simulink model "EPS_MILS"  (R2023a)
settings: Solver=ode23t  StartTime=0.0  StopTime=2  FixedStep=10e-6  RelTol=1e-3
undefined symbols (not defined in the file): Ion, Lithium
libraries: spsSeriesRLCBranchLib x5, spsVoltageMeasurementLib x3, spsPVArrayLib x2, spsCurrentMeasurementLib x2, spsPWMGeneratorDCDCLib x2, spsBatteryLib x1, spsDiodeLib x1, spsIGBTDiodeLib x1, sps_lib x1
settings Model: Creator=Ameya  LastModifiedBy=Ameya

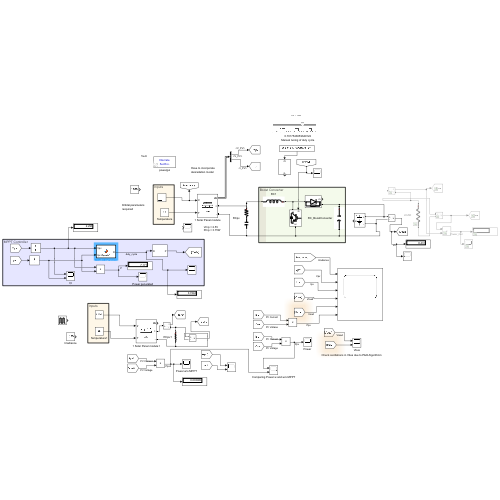
[thumbnail: Simulink's stored preview of the top-level diagram]
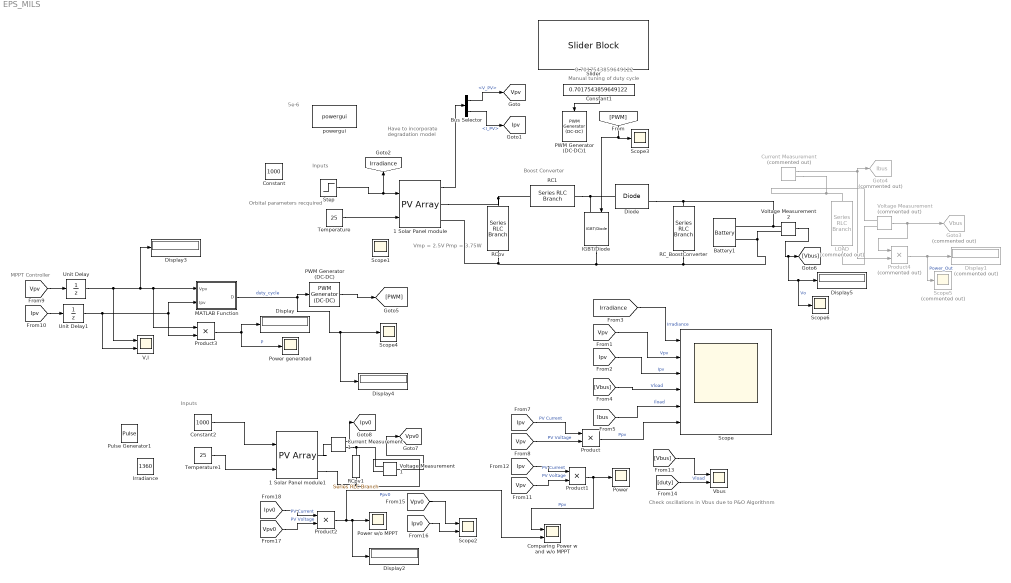
== system EPS_MILS ==
  note: 0.7017543859649122
  note: Manual tuning of duty cycle
  note: Vmp = 2.5V
      | Pmp = 3.75W
  note: 5e-6
  note: Check oscillations in Vbus due to P&O Algorithnm
  note: Boost Converter
  note: Orbital parameters recquired
  note: Have to incorporate degradation model
  note: Inputs
  note: MPPT Controller
  note: Inputs
  1 Solar Panel module : spsPVArrayLib/PV Array  Npar=1  Nser=1  PlotType=one module @ 25 deg.C & specified irradiances  S_vec="[ 1360 1000  500  100 ]"  Temp_C_vec="[ 45 25  ]"  ModuleName=User-defined  PlotWhenSelected=off  Pm=3.75  Ncell=1  Voc=3  Isc=2  Vm=2.5  Im=1.5  beta_Voc_pc=-0.36099  alpha_Isc_pc=0.102  beta_Voc=-0.01083  alpha_Isc=0.00204  IL=2.0248  I0=4.0446e-11  nI=4.7974  Rsh=5.4973  Rs=0.060193  RobustModel=off  RobustCellTemperature=313.3991  BAL=on  Tc=1e-6  Tfilter=5e-5
  1 Solar Panel module1 : spsPVArrayLib/PV Array  Npar=1  Nser=1  PlotType=array @ 25 deg.C & specified irradiances  S_vec="[ 1360 1000  500  100 ]"  Temp_C_vec="[ 45 25  ]"  ModuleName=User-defined  PlotWhenSelected=off  Pm=4.5  Ncell=24  Voc=4  Isc=2  Vm=3  Im=1.5  beta_Voc_pc=-0.3616  alpha_Isc_pc=0.041509  beta_Voc=-0.014464  alpha_Isc=0.00083018  IL=2.0967  I0=5.6287e-11  nI=0.27015  Rsh=6.7146  Rs=0.33348  RobustModel=off  RobustCellTemperature=313.3991  BAL=on  Tc=1e-6  Tfilter=5e-5
  Battery1 : spsBatteryLib/Battery  BatType=Lithium-Ion  ShowTempParam=off  ThermalPreset=no  ShowAgeParam=off  NomV=7.2  NomQ=5.4  SOC=100  Batt_Tr=30  PresetModel=on  MaxQ=5.4  MinV=5.4  FullV=8.3807  Dis_rate=2.3478  R=0.013333  Normal_OP=4.8835  expZone="[7.7788      0.2653]"  current=[6.5 13 32.5]  Units=Time  Tci=20  NomT=20  T2=-30  MaxQ2=4.8  FullV2=7.1  Normal_OP2=5.655  expZone2="[6.58           1]"  Rca=0.6  ti=2000  Dp=0  Neq0=0  Tsim=1e6  Ta1=25  Qeol=5.4*0.9  Reol=0.013333*1.2  Char_age=[2.3478, 3]  Dis_age=[2.3478, 10]  N1=1500  N2=10500  N3=1000  N4=1400  Ta2=45  N5=950
  Bus Selector : BusSelector  OutputSignals=V_PV,I_PV
  Comparing Power w and w/o MPPT : Scope  NumInputPorts=2
  Constant : Constant  Value=1000
  Constant1 : Constant  Value=0.7017543859649122
  Constant2 : Constant  Value=1000
  Current Measurement : spsCurrentMeasurementLib/Current Measurement  Commented=on  PhasorSimulation=off  OutputType=Complex  PSBequivalent=0
  Current Measurement1 : spsCurrentMeasurementLib/Current Measurement  PhasorSimulation=off  OutputType=Complex  PSBequivalent=0
  Diode : spsDiodeLib/Diode  Ron=0.001  Lon=0  Vf=0.8  IC=0  UseSnubber=0  Rs=500  Cs=250e-9  Measurements=on
  Display{,2..5} (5 alike) : Display
  Display1 : Display  Commented=on
  Goto3 : Goto  Commented=on  GotoTag=Vbus  TagVisibility=global
  Goto4 : Goto  Commented=on  GotoTag=Ibus  TagVisibility=global
  IGBT/Diode : spsIGBTDiodeLib/IGBT//Diode  Ron=1e-3  Rs=1e5  Cs=inf  Measurements=off
  Irradiance : Constant  Value=1360
  LOAD : spsSeriesRLCBranchLib/Series RLC Branch  Commented=on  LConnTagsString=__new0  RConnTagsString=__new0  BranchType=R  Resistance=1e-3  Inductance=1e-3  SetiL0=off  InitialCurrent=0  Capacitance=3300e-6  Setx0=off  InitialVoltage=0  Measurements=None
  MATLAB Function : MATLAB Function  TreatAsAtomicUnit=on
  PWM Generator (DC-DC) : spsPWMGeneratorDCDCLib/PWM Generator (DC-DC)  Fsw=5000  Ts=5e-6
  PWM Generator (DC-DC)1 : spsPWMGeneratorDCDCLib/PWM Generator (DC-DC)  Fsw=5000  Ts=5e-6
  "Power " : Scope
  Power generated : Scope
  Power w/o MPPT : Scope
  Product{,1..3} (4 alike) : Product
  Product4 : Product  Commented=on
  Pulse Generator1 : DiscretePulseGenerator  PulseType=Time based  Amplitude=1361  Period=100  PulseWidth=10  PhaseDelay=1
  RC1 : spsSeriesRLCBranchLib/Series RLC Branch  LConnTagsString=__new0  RConnTagsString=__new0  BranchType=L  Resistance=0.1  Inductance=5e-3  SetiL0=off  InitialCurrent=0  Capacitance=5e+3  Setx0=off  InitialVoltage=0  Measurements=None
  RC_BoostConverter : spsSeriesRLCBranchLib/Series RLC Branch  LConnTagsString=__new0  RConnTagsString=__new0  BranchType=C  Resistance=1e-4  Inductance=1e-3  SetiL0=off  InitialCurrent=0  Capacitance=3300e-6  Setx0=off  InitialVoltage=0  Measurements=None
  RCpv : spsSeriesRLCBranchLib/Series RLC Branch  LConnTagsString=__new0  RConnTagsString=__new0  BranchType=RC  Resistance=1e-4  Inductance=1e-3  SetiL0=off  InitialCurrent=0  Capacitance=5e-3  Setx0=off  InitialVoltage=0  Measurements=None
  RCpv1 : spsSeriesRLCBranchLib/Series RLC Branch  LConnTagsString=__new0  RConnTagsString=__new0  BranchType=R  Resistance=1e-3  Inductance=1e-3  SetiL0=off  InitialCurrent=0  Capacitance=5e-3  Setx0=off  InitialVoltage=0  Measurements=None
  Scope : Scope  NumInputPorts=6
  Scope{1,3..4,6} (4 alike) : Scope
  Scope2 : Scope  NumInputPorts=2
  Scope5 : Scope  Commented=on
  Slider : SliderBlock  ScaleMax=1
  Step : Step  Before=1000  After=2000  SampleTime=5e-6
  Temperature : Constant  Value=25
  Temperature1 : Constant  Value=25
  Unit Delay : UnitDelay  SampleTime=-1  HasFrameUpgradeWarning=on
  Unit Delay1 : UnitDelay  SampleTime=-1  HasFrameUpgradeWarning=on
  V,I : Scope  NumInputPorts=2
  Vbus : Scope  NumInputPorts=2
  Voltage Measurement : spsVoltageMeasurementLib/Voltage Measurement  Commented=on  PhasorSimulation=off  OutputType=Complex  PSBequivalent=0
  Voltage Measurement1 : spsVoltageMeasurementLib/Voltage Measurement  PhasorSimulation=off  OutputType=Complex  PSBequivalent=0
  Voltage Measurement2 : spsVoltageMeasurementLib/Voltage Measurement  PhasorSimulation=off  OutputType=Complex  PSBequivalent=0
  powergui : sps_lib/powergui  Priority=1  SimulationMode=Discrete  SampleTime=5e-6  frequency=60  Iterations=50  frequencyindice=0  Pbase=100e6  ErrMax=1e-4  UnitsV=kV  UnitsW=MW  buscounter=0  FunctionMessages=off  echomessages=off  EnableUseOfTLC=off  CurrentSourceSwitches=off  DisableSnubberDevices=off  DisableRonSwitches=off  DisableVfSwitches=off  DisplayEquations=off  AutomaticDiscreteSolvers=off  SolverType=Tustin/Backward Euler (TBE)  Interpol=off  ExternalGateDelay=off  methode=off  Ts=100  x0status=blocks  SPID=on  SwTol=0  HookPort=off  NonlinearTolerance=1e-4  nMaxIteration=100  ContinueOnMaxIteration=off  RestoreLinks=warning  ResistiveCurrentMeasurement=off  Frange=[0:2:500]  Ylog=off  Xlog=on  ShowGrid=off  save=off  variable=ZData  structure=0  ZoomFFT=off  StartTime=0.0  cycles=1  DisplayStyle=1  fundamental=60  FreqAxis=off  MaxFrequency=1000  frequencyindicesteady=1  RmsSteady=1  display=off
  tag scope: Ipv0=global, Ipv=global, Irradiance=global, Vpv0=global, Vpv=global
  wires:
  1 Solar Panel module/1 -> Bus Selector/1
  Bus Selector/1 -> [Vpv]  "<V_PV>"
  Bus Selector/2 -> [Ipv]  "<I_PV>"
  Temperature/1 -> 1 Solar Panel module/2
  Voltage Measurement/1 -> Product4/1, Goto3/1
  Current Measurement/1 -> Goto4/1, Product4/2
  [Irradiance] -> Scope/1  "Irradiance"
  [Vpv] -> Scope/2  "Vpv"
  [Ipv] -> Scope/3  "Ipv"
  [Vbus] -> Scope/4  "Vload"
  [Ibus] -> Scope/5  "Iload"
  Product/1 -> Scope/6  "Ppv"
  [Ipv] -> Product/1  "PV Current"
  [Vpv] -> Product/2  "PV Voltage"
  PWM Generator (DC-DC)/1 -> [PWM]
  MATLAB Function/1(D) -> Display4/1, Scope4/1, PWM Generator (DC-DC)/1  "duty_cycle"
  [Vpv] -> Unit Delay/1
  [Ipv] -> Unit Delay1/1
  [Vpv] -> Product1/2  "PV Voltage"
  Product1/1 -> Comparing Power w and w/o MPPT/1, "Power "/1  "Ppv"
  [Ipv] -> Product1/1  "PV Current"
  [Vbus] -> Vbus/1  "Vload"
  [duty] -> Vbus/2
  Temperature1/1 -> 1 Solar Panel module1/2
  [Vpv0] -> Scope2/1
  [Ipv0] -> Scope2/2
  Voltage Measurement1/1 -> [Vpv0]
  Current Measurement1/1 -> [Ipv0]
  [Vpv0] -> Product2/2  "PV Voltage"
  [Ipv0] -> Product2/1  "PV Current"
  Product2/1 -> Comparing Power w and w/o MPPT/2, Display2/1, Power w/o MPPT/1  "Ppv0"
  Product3/1 -> Power generated/1, Display/1  "P"
  Product4/1 -> Scope5/1, Display1/1  "Power_Out"
  Constant1/1 -> PWM Generator (DC-DC)1/1
  [PWM] -> IGBT/Diode/1, Scope3/1
  Unit Delay/1 -> V,I/1, Display3/1, Product3/1, MATLAB Function/1(Vpv)
  Unit Delay1/1 -> V,I/2, Product3/2, MATLAB Function/2(Ipv)
  Constant2/1 -> 1 Solar Panel module1/1
  Voltage Measurement2/1 -> Scope6/1, Display5/1, [Vbus]  "Vo"
  Step/1 -> [Irradiance], 1 Solar Panel module/1
  connections:
  1 Solar Panel module/RConn1 -- RC1/RConn1 -- RCpv/LConn1
  RCpv/RConn1 -- Battery1/LConn2 -- Voltage Measurement2/LConn2 -- RC_BoostConverter/RConn1 -- IGBT/Diode/RConn1 -- 1 Solar Panel module/RConn2
  RC1/LConn1 -- Diode/LConn1 -- IGBT/Diode/LConn1
  Diode/RConn1 -- RC_BoostConverter/LConn1 -- Battery1/LConn1 -- Voltage Measurement2/LConn1
  LOAD/LConn1 -- Voltage Measurement/LConn1 -- Current Measurement/RConn1
  Voltage Measurement1/LConn1 -- RCpv1/LConn1 -- Current Measurement1/RConn1
  1 Solar Panel module1/RConn2 -- Voltage Measurement1/LConn2 -- RCpv1/RConn1
  1 Solar Panel module1/RConn1 -- Current Measurement1/LConn1
  Voltage Measurement/LConn2 -- LOAD/RConn1

== matlab function EPS_MILS/MATLAB Function ==
  data: Vpv input; D output; Ipv input
function D = PandO(Vpv,Ipv)
%Duty Cycle is the ratio of the pulse width to the time period
Dmin = 0;
Dmax = 1;
Dinit = 0.7;

%Solar cell parameters
Voc = 4
Isc = 2
Vmp = 2.5
Pmp = 3.75

    persistent Dprev Pprev Vprev;
    if isempty(Dprev)
        Dprev = Dinit;
        Pprev = 0;
        Vprev = 0;
    end
    
    %Boost Converter Vo/Vi = 1/(1-D)
    %Keeping Vo constant we are trying to maintaing Vi=Vmp
    %Vi = (1-D)*Vo
    

    %Calulating Power
    Ppv = Ipv*Vpv;
    dP = Ppv-Pprev;
    dV = Vpv -Vprev;

    deltaD = 1e-6;
    
    if dP ~= 0
        if dP>0
            if dV>0
                D = Dprev - deltaD;
            else
                D = Dprev + deltaD;
            end
        else
            if dV>0
                D = Dprev + deltaD;
            else
                D = Dprev - deltaD;
            end
        end
    else
        D = Dprev;
    end
    
    %D should be forced to be between 0 and 1, Its going below 0
    if D>Dmax||D<Dmin
        D=Dprev;
    end

    %Updating internal values
    Dprev = D;
    Vprev = Vpv;
    Pprev = Ppv;
end
